simulink model "q_rotpen_swingup_student"  (R2020a)
settings: Solver=ode1  StartTime=0.0  StopTime=inf  FixedStep=0.002  RelTol=1e-3  EnableMultiTasking=on
PostLoadFcn:
  | qc_set_target_type(getConfigSet(bdroot, 'QUARC Default Target Configuration'));
values from neighbouring files (symbols this model uses):
  a_max = T_max/(Mr*Lr)    (= 11.5752306332)    [Furuta_Pedulum.m]
  epsilon = 12.0 * pi / 180    (= 0.209439510239)    [Furuta_Pedulum.m]
  Er = Ep_upright_position    [Furuta_Pedulum.m]
  K_AMP = 1    [Furuta_Pedulum.m]
  K_ENC = 2 * pi / ( 4 * 1024 )    (= 0.00153398078789)    [Furuta_Pedulum.m]
  wcf_1 = 2 * pi * 10.0    (= 62.8318530718)    [Furuta_Pedulum.m]
  wcf_2 = 2 * pi * 10.0    (= 62.8318530718)    [Furuta_Pedulum.m]
undefined symbols (not defined in the file or in its folder): HIL, K, qc_get_step_size
libraries: simulink_extras x3, simulink x3, quarc_library x3
settings Model: SimulationMode=external  ExtModeTrigDuration=10000  Creator=MLevis  LastModifiedBy=mathe
settings SolverCC: PositivePriorityOrder=on
settings DataIOCC: LimitDataPoints=on  SaveFormat=Array  SignalLoggingSaveFormat=ModelDataLogs  ReturnWorkspaceOutputs=off
settings OptimizationCC: ExpressionDepthLimit=2147483647  InitFltsAndDblsToZero=on  LifeSpan=inf
settings DebuggingCC: SaveWithParameterizedLinksMsg=none  UnderspecifiedInitializationDetection=Classic  MergeDetectMultiDrivingBlocksExec=none  SolverPrmCheckMsg=warning  MultiTaskDSMMsg=warning  MultiTaskCondExecSysMsg=none  FcnCallInpInsideContextMsg=warning  StateNameClashWarn=warning  SFUnexpectedBacktrackingDiag=warning  SFNoUnconditionalDefaultTransitionDiag=warning  SFExecutionAtInitializationDiag=none  ArithmeticOperatorsInVariantConditions=warning
settings HardwareCC: ProdBitPerPointer=32  ProdBitPerSizeT=32  ProdBitPerPtrDiffT=32  ProdLargestAtomicFloat=None  ProdIntDivRoundTo=Undefined  ProdEndianess=Unspecified  ProdWordSize=32  ProdHWDeviceType=32-bit Generic
settings ModelReferenceCC: PropagateSignalLabelsOutOfModel=off
settings SFSimCC: SimUseLocalCustomCode=off  CustomCodeUndefinedFunction=UseInterfaceOnly
settings RTWCC: Description=QUARC Win64 Target  SystemTargetFile=quarc_win64.tlc  TemplateMakefile=quarc_default_tmf  RTWUseLocalCustomCode=off
settings CodeAppCC: StateflowObjectComments=on
settings STFCustomTargetCC: TargetPreCompLibLocation=C:\PROGRA~3\QUARC\lib\2018b\win64\release  CPPClassGenCompliant=on  GRTInterface=on  SystemTargetFile=quarc_win64.tlc
settings GRTTargetCC: TargetPreCompLibLocation=C:\PROGRA~3\QUARC\lib\2018b\win64\release  TargetLangStandard=C89/C90 (ANSI)  ParMdlRefBuildCompliant=off  CompOptLevelCompliant=off  ConcurrentExecutionCompliant=off  CombineOutputUpdateFcns=off  MatFileLogging=off  GRTInterface=on  UseToolchainInfoCompliant=off  ExtMode=on  ExtModeMexFile=quarc_comm
settings ConfigComp: CovMetricSettings=dw  CovHtmlReporting=on  CovSaveCumulativeToWorkspaceVar=on  CovSaveSingleToWorkspaceVar=on  CovExternalEMLEnable=off

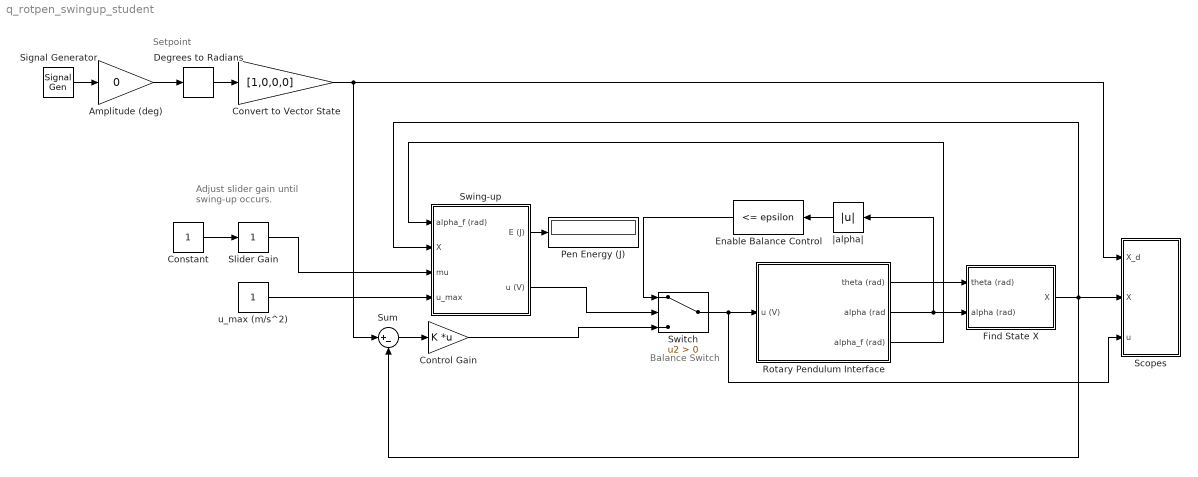
== system q_rotpen_swingup_student ==
  note: Balance Switch
  note: Setpoint
  note: Adjust slider gain
      | until swing-up occurs.
  Amplitude (deg) : Gain  Gain=0  SaturateOnIntegerOverflow=on  OutDataTypeStr=Inherit: Same as input  ParamDataTypeStr=Inherit: Same as input
  Constant : Constant
  Control Gain : Gain  Gain=K  Multiplication=Matrix(K*u)
  Convert to Vector State : Gain  Gain=[1,0,0,0]
  Degrees to Radians : simulink_extras/Transformations/Degrees to Radians
  Enable Balance Control : simulink/Logic and Bit Operations/Compare To Constant  relop=<=  const=epsilon  OutDataTypeStr=uint8  ZeroCross=off
  Find State X : Subsystem
  Pen Energy (J) : Display
      settings: Decimation=100
  Rotary Pendulum Interface : Subsystem
  Scopes : Subsystem
  Signal Generator : SignalGenerator  WaveForm=square  Frequency=0.1
  Slider Gain : simulink/Math Operations/Slider Gain  gain=1  low=0  high=10
  Sum : Sum  Inputs=|+-
  Swing-up : Subsystem
  Switch : Switch  Criteria=u2 > Threshold
  u_max (m/s^2) : Constant
  |alpha| : Abs
  wires:
  Amplitude (deg)/1 -> Degrees to Radians/1
  Signal Generator/1 -> Amplitude (deg)/1
  Degrees to Radians/1 -> Convert to Vector State/1
  Convert to Vector State/1 -> Scopes/1(X_d), Sum/1
  Find State X/1(X) -> Scopes/2(X), Sum/2, Swing-up/2(X)
  Rotary Pendulum Interface/1(theta (rad)) -> Find State X/1(theta (rad))
  Rotary Pendulum Interface/2(alpha (rad) -> Find State X/2(alpha (rad)), |alpha|/1
  Sum/1 -> Control Gain/1
  Switch/1 -> Rotary Pendulum Interface/1(u (V)), Scopes/3(u)
  |alpha|/1 -> Enable Balance Control/1
  Rotary Pendulum Interface/3(alpha_f (rad)) -> Swing-up/1(alpha_f (rad))
  Constant/1 -> Slider Gain/1
  Slider Gain/1 -> Swing-up/3(mu)
  Swing-up/1(E (J)) -> Pen Energy (J)/1
  u_max (m/s^2)/1 -> Swing-up/4(u_max)
  Enable Balance Control/1 -> Switch/1
  Swing-up/2(u (V)) -> Switch/2
  Control Gain/1 -> Switch/3

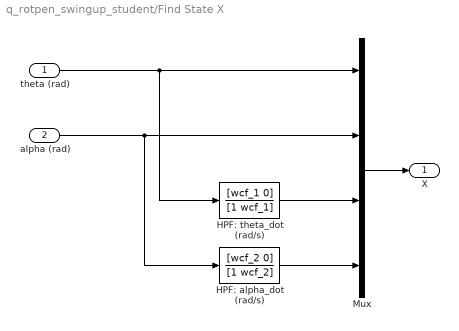
== system q_rotpen_swingup_student/Find State X ==
  theta (rad) : Inport
  alpha (rad) : Inport  Port=2
  HPF: alpha_dot (rad/s) : TransferFcn  Numerator=[wcf_2 0]  Denominator=[1 wcf_2]
  HPF: theta_dot (rad/s) : TransferFcn  Numerator=[wcf_1 0]  Denominator=[1 wcf_1]
  Mux : Mux
  X : Outport  VectorParamsAs1DForOutWhenUnconnected=off
  wires:
  alpha (rad)/1 -> Mux/2, HPF: alpha_dot (rad/s)/1
  Mux/1 -> X/1
  theta (rad)/1 -> Mux/1, HPF: theta_dot (rad/s)/1
  HPF: theta_dot (rad/s)/1 -> Mux/3
  HPF: alpha_dot (rad/s)/1 -> Mux/4

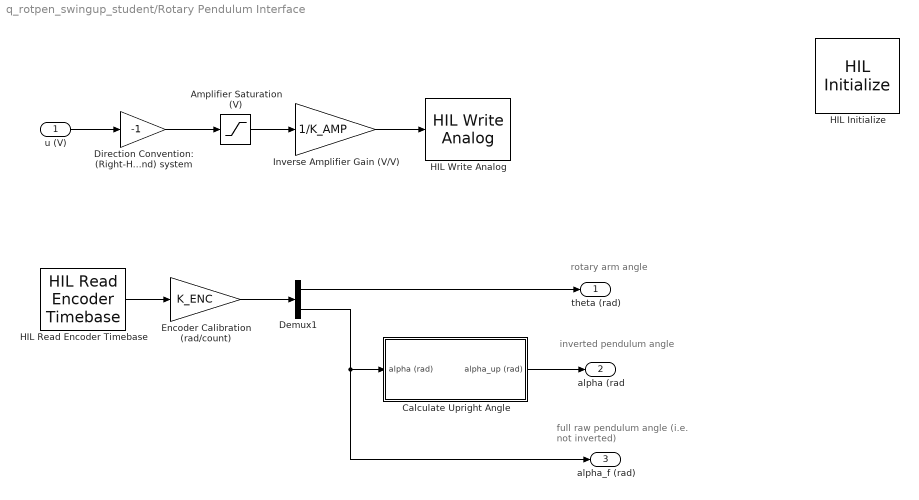
== system q_rotpen_swingup_student/Rotary Pendulum Interface ==
  note: full raw pendulum angle
      |  (i.e. not inverted)
  note: rotary arm angle
  note: inverted pendulum angle
  u (V) : Inport
  Amplifier Saturation (V) : Saturate  UpperLimit=5  LowerLimit=-5
  Calculate Upright Angle : Subsystem
  Demux1 : Demux  Outputs=2
  Direction Convention: (Right-Hand) system : Gain  Gain=-1  SaturateOnIntegerOverflow=on  OutDataTypeStr=Inherit: Same as input  ParamDataTypeStr=Inherit: Same as input
  Encoder Calibration (rad/count) : Gain  Gain=K_ENC  SaturateOnIntegerOverflow=on  OutDataTypeStr=Inherit: Same as input  ParamDataTypeStr=Inherit: Same as input
  HIL Initialize : quarc_library/Data Acquisition/Generic/Configuration/HIL Initialize  object_name=HIL-1  board_type=q2_usb  board_number=0  board_options=d0=digital;d1=digital;led=auto;update_rate=normal;decimation=1  exclusive=off  active=off  hardware_clocks=[0]  clock_modes=[]  initial_clock_frequencies=[]  set_clock_params_at_start=off  set_clock_params_at_switch_in=off  set_clock_frequencies_at_start=off  set_clock_frequencies_at_switch_in=off  analog_input_channels=[0:1]  analog_input_configurations=[]  analog_input_maximums=10  analog_input_minimums=-10  set_analog_input_params_at_start=on  set_analog_input_params_at_switch_in=off  analog_output_channels=[0:1]  analog_output_maximums=10  analog_output_minimums=-10  initial_analog_outputs=[0]  final_analog_outputs=[0]  watchdog_analog_outputs=0  set_analog_output_params_at_start=on  set_analog_output_params_at_switch_in=off  set_analog_outputs_at_start=on  set_analog_outputs_at_switch_in=off  set_analog_outputs_at_terminate=on  set_analog_outputs_at_switch_out=off  set_analog_outputs_on_watchdog=off  digital_input_channels=[]  digital_output_channels=[]  digital_output_configuration=[]  initial_digital_outputs=[1]  final_digital_outputs=[1]  watchdog_digital_outputs=[1]  set_digital_output_params_at_start=off  set_digital_output_params_at_switch_in=off  set_digital_outputs_at_start=on  set_digital_outputs_at_switch_in=off  set_digital_outputs_at_terminate=on  set_digital_outputs_at_switch_out=off  set_digital_outputs_on_watchdog=off  encoder_channels=[0:1]  quadrature=[4]  encoder_filter_frequency=[]  initial_encoder_counts=[0]  set_encoder_params_at_start=on  set_encoder_params_at_switch_in=off  set_encoder_counts_at_start=on  set_encoder_counts_at_switch_in=off  pwm_channels=[]  pwm_modes=[0]  pwm_frequency=1/0.020  pwm_configuration=[]  pwm_alignment=[]  pwm_polarity=[]  pwm_leading_deadband=[]  pwm_trailing_deadband=[]  initial_pwm_outputs=[0]  final_pwm_outputs=[0]  watchdog_pwm_outputs=[0]  set_pwm_params_at_start=on  set_pwm_params_at_switch_in=off  set_pwm_outputs_at_start=on  set_pwm_outputs_at_switch_in=off  set_pwm_outputs_at_terminate=on  set_pwm_outputs_at_switch_out=off  set_pwm_outputs_on_watchdog=off  other_output_channels=[]  initial_other_outputs=[]  final_other_outputs=[]  watchdog_other_outputs=[]  set_other_outputs_at_start=off  set_other_outputs_at_switch_in=off  set_other_outputs_at_terminate=off  set_other_outputs_at_switch_out=off  set_other_outputs_on_watchdog=off
  HIL Read Encoder Timebase : quarc_library/Data Acquisition/Generic/Timebases/HIL Read Encoder Timebase  object_name=HIL-1  clock=0  channels=[0:1]  samples_in_buffer=max(ceil(1/qc_get_step_size), 1)  active=on  vector_output=on  data_type_mode=Inherit via back propagation  data_type=double
  HIL Write Analog : quarc_library/Data Acquisition/Generic/Immediate I//O/HIL Write Analog  object_name=HIL-1  channels=0  sample_time=-1  active=off  vector_input=off
  Inverse Amplifier Gain (V/V) : Gain  Gain=1/K_AMP
  theta (rad) : Outport  VectorParamsAs1DForOutWhenUnconnected=off
  alpha (rad : Outport  Port=2  VectorParamsAs1DForOutWhenUnconnected=off
  alpha_f (rad) : Outport  Port=3  VectorParamsAs1DForOutWhenUnconnected=off
  wires:
  Calculate Upright Angle/1(alpha_up (rad)) -> alpha (rad/1
  Demux1/1 -> theta (rad)/1
  Direction Convention: (Right-Hand) system/1 -> Amplifier Saturation (V)/1
  u (V)/1 -> Direction Convention: (Right-Hand) system/1
  Inverse Amplifier Gain (V/V)/1 -> HIL Write Analog/1
  Amplifier Saturation (V)/1 -> Inverse Amplifier Gain (V/V)/1
  HIL Read Encoder Timebase/1 -> Encoder Calibration (rad/count)/1
  Demux1/2 -> alpha_f (rad)/1, Calculate Upright Angle/1(alpha (rad))
  Encoder Calibration (rad/count)/1 -> Demux1/1

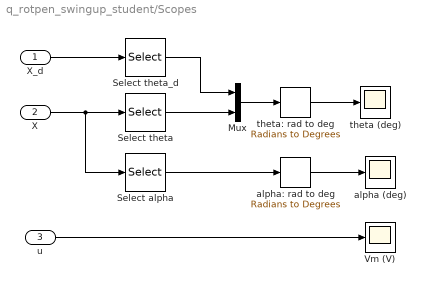
== system q_rotpen_swingup_student/Scopes ==
  X_d : Inport
  X : Inport  Port=2
  u : Inport  Port=3
  Mux : Mux  Inputs=2
  Select alpha : Selector  InputPortWidth=4  IndexOptions=Index vector (dialog)  Indices=2  OutputSizes=[(-2)]
  Select theta : Selector  InputPortWidth=4  IndexOptions=Index vector (dialog)  Indices=1  OutputSizes=[(-2)]
  Select theta_d : Selector  InputPortWidth=4  IndexOptions=Index vector (dialog)  Indices=1  OutputSizes=[(-2)]
  Vm (V) : Scope
  alpha (deg) : Scope
  alpha: rad to deg : simulink_extras/Transformations/Radians to Degrees
  theta (deg) : Scope
  theta: rad to deg : simulink_extras/Transformations/Radians to Degrees
  wires:
  u/1 -> Vm (V)/1
  X_d/1 -> Select theta_d/1
  Mux/1 -> theta: rad to deg/1
  Select alpha/1 -> alpha: rad to deg/1
  alpha: rad to deg/1 -> alpha (deg)/1
  X/1 -> Select alpha/1, Select theta/1
  Select theta_d/1 -> Mux/1
  theta: rad to deg/1 -> theta (deg)/1
  Select theta/1 -> Mux/2

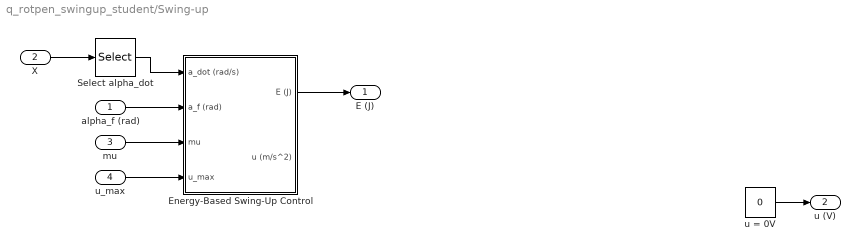
== system q_rotpen_swingup_student/Swing-up ==
  alpha_f (rad) : Inport
  X : Inport  Port=2
  mu : Inport  Port=3
  u_max : Inport  Port=4
  Energy-Based Swing-Up Control : Subsystem
  Select alpha_dot : Selector  InputPortWidth=4  IndexOptions=Index vector (dialog)  Indices=[4]  OutputSizes=1
  u = 0V : Constant  Value=0
  E (J) : Outport  VectorParamsAs1DForOutWhenUnconnected=off
  u (V) : Outport  Port=2  VectorParamsAs1DForOutWhenUnconnected=off
  wires:
  Energy-Based Swing-Up Control/1(E (J)) -> E (J)/1
  alpha_f (rad)/1 -> Energy-Based Swing-Up Control/2(a_f (rad))
  mu/1 -> Energy-Based Swing-Up Control/3(mu)
  Select alpha_dot/1 -> Energy-Based Swing-Up Control/1(a_dot (rad/s))
  X/1 -> Select alpha_dot/1
  u_max/1 -> Energy-Based Swing-Up Control/4(u_max)
  u = 0V/1 -> u (V)/1

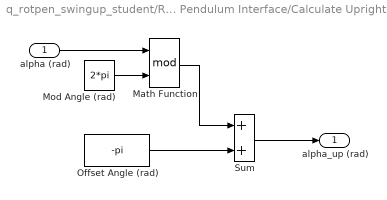
== system q_rotpen_swingup_student/Rotary Pendulum Interface/Calculate Upright Angle ==
  alpha (rad) : Inport
  Math Function : Math  Operator=mod  SignedPower=on  SaturateOnIntegerOverflow=on
  Mod Angle (rad) : Constant  Value=2*pi
  Offset Angle (rad) : Constant  Value=-pi
  Sum : Sum  InputSameDT=on  SaturateOnIntegerOverflow=on  OutDataTypeStr=Inherit: Same as first input
  alpha_up (rad) : Outport  VectorParamsAs1DForOutWhenUnconnected=off
  wires:
  Math Function/1 -> Sum/1
  alpha (rad)/1 -> Math Function/1
  Offset Angle (rad)/1 -> Sum/2
  Mod Angle (rad)/1 -> Math Function/2
  Sum/1 -> alpha_up (rad)/1

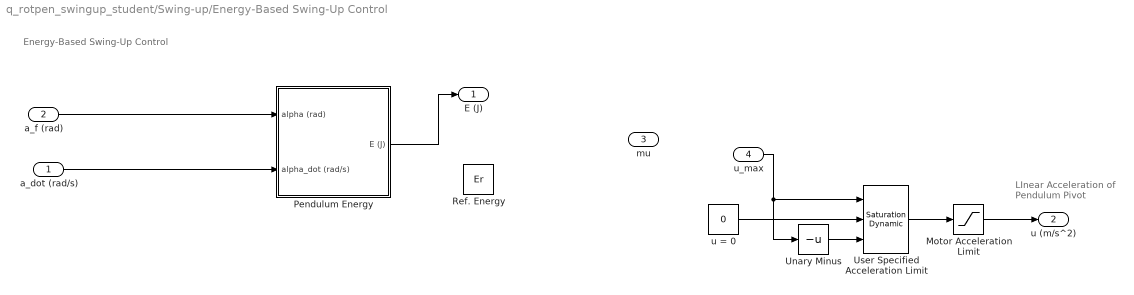
== system q_rotpen_swingup_student/Swing-up/Energy-Based Swing-Up Control ==
  note: Energy-Based Swing-Up Control
  note: LInear Acceleration of
      | Pendulum Pivot
  a_dot (rad/s) : Inport
  a_f (rad) : Inport  Port=2
  mu : Inport  Port=3
  u_max : Inport  Port=4
  Motor Acceleration Limit : Saturate  UpperLimit=a_max  LowerLimit=-a_max
  Pendulum Energy : Subsystem
  Ref. Energy : Constant  Value=Er
  Unary Minus : UnaryMinus
  User Specified Acceleration Limit : simulink/Discontinuities/Saturation Dynamic  OutMin=[]  OutMax=[]  OutDataTypeStr=Inherit: Same as second input  OutDataType=fixdt(1, 16)  OutScaling=2^-10  DoSatur=off
  u = 0 : Constant  Value=0
  E (J) : Outport  VectorParamsAs1DForOutWhenUnconnected=off
  u (m/s^2) : Outport  Port=2  VectorParamsAs1DForOutWhenUnconnected=off
  wires:
  a_f (rad)/1 -> Pendulum Energy/1(alpha (rad))
  Pendulum Energy/1(E (J)) -> E (J)/1
  a_dot (rad/s)/1 -> Pendulum Energy/2(alpha_dot (rad/s))
  u = 0/1 -> User Specified Acceleration Limit/2
  u_max/1 -> User Specified Acceleration Limit/1, Unary Minus/1
  Unary Minus/1 -> User Specified Acceleration Limit/3
  User Specified Acceleration Limit/1 -> Motor Acceleration Limit/1
  Motor Acceleration Limit/1 -> u (m/s^2)/1

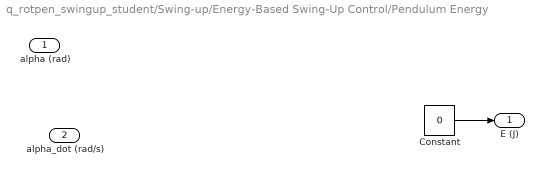
== system q_rotpen_swingup_student/Swing-up/Energy-Based Swing-Up Control/Pendulum Energy ==
  alpha (rad) : Inport
  alpha_dot (rad/s) : Inport  Port=2
  Constant : Constant  Value=0
  E (J) : Outport  VectorParamsAs1DForOutWhenUnconnected=off
  wires:
  Constant/1 -> E (J)/1
